simulink model "angle_control_check"  (R2024a)
settings: Solver=ode1  StartTime=0.0  StopTime=inf  FixedStep=1/60  RelTol=1e-3  EnableMultiTasking=on
model workspace (MAT data in the model file):
  downCamStepSize : Simulink.Parameter (value not decoded)
  lidarStepSize : Simulink.Parameter (value not decoded)
  mainStepSize : Simulink.Parameter (value not decoded)
  mode : Simulink.Parameter (value not decoded)
  realSenseStepSize : Simulink.Parameter (value not decoded)
symbols that are objects in the model workspace (value not decoded): downCamStepSize, lidarStepSize, mainStepSize, realSenseStepSize
undefined symbols (not defined in the file): gcbh, JPEG, Point, video_display_show
libraries: quarc_library x33, simulink x3
(part 2 of 2)

== matlab function angle_control_check/QBot Hardware/Differential Drive Forward Velocity Kinematics ==
  data: wL input; vC output; wR input; Omega output
function [vC , Omega] = forKin(wL, wR)

% calculate wheel angular velocities
wheelRadius = 3.5*0.0254/2;

vR = wR * wheelRadius;
vL = wL * wheelRadius;

% wheelbase
d=0.3928; 

% calculate wheel linear velocities
vC = (vR + vL)/2;
Omega = (vR - vL)/d;

== matlab function angle_control_check/Lidar & Localization/Adjust for Center of Measurement ==
  data: lidar_position input; ranges input; ranges_c output; angles input; angles_c output
function [ranges_c,angles_c] = correct_lidar(lidar_position, ranges,angles)

% Convert lidar data from polar into cartesian, and add lidar position
x = ranges.*cos(angles) + lidar_position(1);
y = ranges.*sin(angles) + lidar_position(2);

% Convert back into polar coordinates
ranges_c = sqrt(x.^2 + y.^2);
angles_c = atan2(y, x);

end

== matlab function angle_control_check/Image Processing (Line Following)/colorize ==
  data: Binary input; y output; Color input
function y = fcn(Binary, Color)

y = Color;
[ROW, COL, ~] = size(y);

y(51:100, 1:COL, 1) = ((255 - Binary)/255).*Color(51:100,:,1) + (Binary).*Color(51:100, :, 1);
y(51:100, 1:COL, 2) = ((255 - Binary)/255).*Color(51:100,:,2);
y(51:100, 1:COL, 3) = ((255 - Binary)/255).*Color(51:100,:,3);
